simulink model "Boiler_autom"  (R2021b)
settings: Solver=FixedStepAuto  StartTime=0.0  StopTime=20  FixedStep=0.01  RelTol=1e-3
settings Model: Creator=Falk  LastModifiedBy=Falk
settings DataIOCC: InspectSignalLogs=on

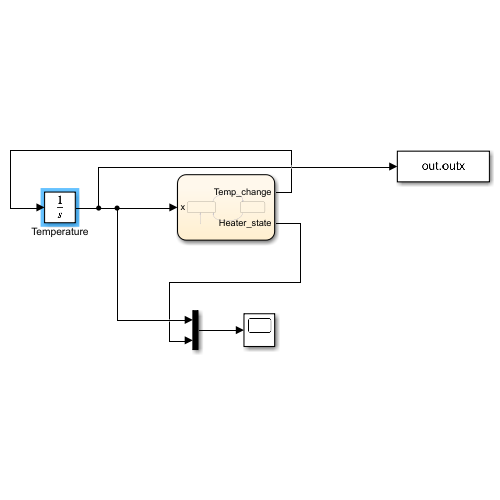
[thumbnail: Simulink's stored preview of the top-level diagram]
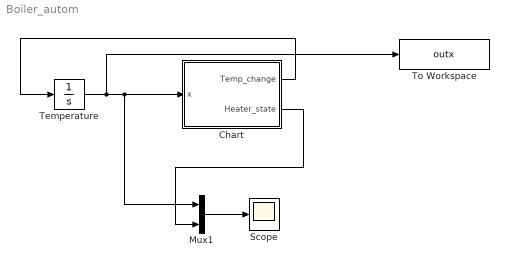
== system Boiler_autom ==
  Chart : Stateflow chart  TreatAsAtomicUnit=on
  Mux1 : Mux  Inputs=2
  Scope : Scope
  Temperature : Integrator  InitialCondition=15
  To Workspace : ToWorkspace  VariableName=outx  SampleTime=-1
  wires:
  Mux1/1 -> Scope/1
  Chart/2(Heater_state) -> Mux1/2
  Chart/1(Temp_change) -> Temperature/1
  Temperature/1 -> To Workspace/1, Mux1/1, Chart/1(x)

== stateflow chart Boiler_autom/Chart ==
  state t1
    Temp_change = 0.5*x+0.5;
    Heater_state = 1;
  state t3
    Temp_change = -0.5*x;
    Heater_state = 0;
  t1 -> t3 : [x >= 25]
  (default) -> t1
  t3 -> t1 : [x <= 20]
  data: x input; Temp_change output; Heater_state output
